simulink model "BMS_test"  (R2022b)
settings: Solver=FixedStepAuto  StartTime=0.0  StopTime=inf  FixedStep=0.005  RelTol=1e-3
undefined symbols (not defined in the file): canChannel
libraries: canlib x3, canmsglib x2, battery_monitor_lib x1
settings Model: Creator=LinF  LastModifiedBy=LinF

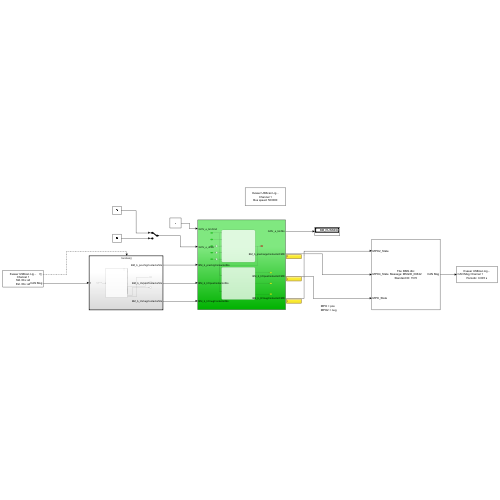
[thumbnail: Simulink's stored preview of the top-level diagram]
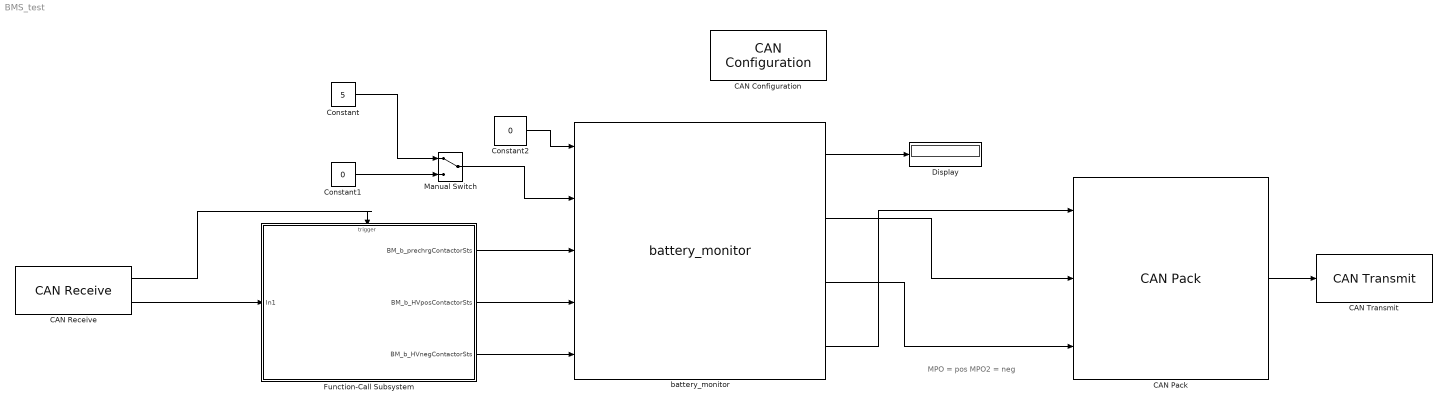
== system BMS_test ==
  note: MPO = pos
      | MPO2 = neg
  CAN Configuration : canlib/CAN Configuration  BlockHandle=2.0897  Device=Kvaser USBcan Light 1 (Channel 1)  DeviceMenu=Kvaser USBcan Light 1 (Channel 1)  ObjConstructor=canChannel('Kvaser', 'USBcan Light 1', 1)  BusSpeed=500000  EnableBitParameters=off  SJW=1  TSEG1=4  TSEG2=3  NSamples=1  AckMode=Normal
  CAN Pack : canmsglib/CAN Pack  CANdbFile=C:\Users\LinF\Documents\MACFE\Embedded\CAN_Databases\BMS.dbc  MsgList=MSGID_0X622  MsgName=MSGID_0X622  MsgIDType=Standard (11-bit identifier)  MsgIdentifier=1570  MsgLength=3  Remote=off  ApplyMinMax=off  BusOutput=off  SignalInfo={'MPO2_State','16','8','BE','unsigned','Standard','0','1','0','-Inf','Inf';'MPO4_State','8','8','BE','unsigned','Standard','0','1','0','-Inf','Inf';'MPO_State','0','8','BE','unsigned','Standard','0','1','0','-Inf','Inf'}
      settings: LibrarySourceBlock=embeddedtargetslib/Host Communication/CAN Pack  DataFormat=CANdb specified signals
  CAN Receive : canlib/CAN Receive  BlockHandle=8.0004  Device=Kvaser USBcan Light 1 (Channel 1)  DeviceMenu=Kvaser USBcan Light 1 (Channel 1)  ObjConstructor=canChannel('Kvaser', 'USBcan Light 1', 1)  EnableStandardIDsFilter=off  StdIDsCombo=Allow all  StandardIDs=0  EnableExtendedIDsFilter=off  ExtIDsCombo=Allow all  ExtendedIDs=0  SampleTime=0.005  MsgsPerTimestep=all  InternalFilterUpdateStatus=on  BusOutput=off
  CAN Transmit : canlib/CAN Transmit  BlockHandle=11.0004  Device=Kvaser USBcan Light 1 (Channel 1)  DeviceMenu=Kvaser USBcan Light 1 (Channel 1)  ObjConstructor=canChannel('Kvaser', 'USBcan Light 1', 1)  EnableEventTransmit=off  EnablePeriodicTransmit=on  MessagePeriod=0.005
  Constant : Constant  Value=5
  Constant1 : Constant  Value=0
  Constant2 : Constant  Value=0
  Display : Display
  Function-Call Subsystem : Subsystem  TreatAsAtomicUnit=on
  Manual Switch : ManualSwitch
  battery_monitor : battery_monitor_lib/battery_monitor  SystemSampleTime=-1  VariantActivationTime=update diagram  Latency=0  AutoFrameSizeCalculation=off
  wires:
  Manual Switch/1 -> battery_monitor/2
  Constant/1 -> Manual Switch/1
  Constant1/1 -> Manual Switch/2
  battery_monitor/1 -> Display/1
  Constant2/1 -> battery_monitor/1
  CAN Receive/2 -> Function-Call Subsystem/1(In1)
  CAN Receive/1 -> Function-Call Subsystem/Trigger
  battery_monitor/3 -> CAN Pack/3
  battery_monitor/4 -> CAN Pack/1
  battery_monitor/2 -> CAN Pack/2
  CAN Pack/1 -> CAN Transmit/1
  Function-Call Subsystem/1(BM_b_prechrgContactorSts) -> battery_monitor/3
  Function-Call Subsystem/2(BM_b_HVposContactorSts) -> battery_monitor/4
  Function-Call Subsystem/3(BM_b_HVnegContactorSts) -> battery_monitor/5

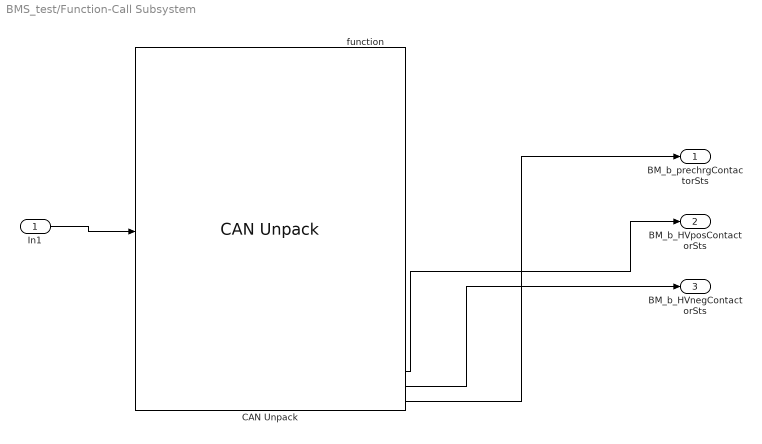
== system BMS_test/Function-Call Subsystem ==
  In1 : Inport
  function : TriggerPort  TriggerType=function-call  VariantControl=(inherit)
  CAN Unpack : canmsglib/CAN Unpack  CANdbFile=C:\Users\LinF\Documents\MACFE\Embedded\CAN_Databases\BMS.dbc  MsgList=MSGID_0X626  MsgName=MSGID_0X626  MsgIDType=Standard (11-bit identifier)  MsgIdentifier=1574  MsgLength=3  SignalInfo={'Blank','1','1','LE','unsigned','Standard','0','1','0','0','1';'Blank','2','1','LE','unsigned','Standard','0','1','0','0','1';'Blank','3','1','LE','unsigned','Standard','0','1','0','0','1';'Blank','4','1','LE','unsigned','Standard','0','1','0','0','1';'Blank','5','1','LE','unsigned','Standard','0','1','0','0','1';'Blank','6','1','LE','unsigned','Standard','0','1','0','0','1';'Blank','7','1','LE','unsigned','Standard','0','1','0','0','1';'Blank','9','1','LE','unsigned','Standard','0','1','0','0','1';'Blank','10','1','LE','unsigned','Standard','0','1','0','0','1';'Blank','11','1','LE','unsigned','Standard','0','1','0','0','1';'Blank','12','1','LE','unsigned','Standard','0','1','0','0','1';'Blank','13','1','LE','unsigned','Standard','0','1','0','0','1';'Blank','14','1','LE','unsigned','Standard','0','1','0','0','1';'Blank','15','1','LE','unsigned','Standard','0','1','0','0','1';'Blank','17','1','LE','unsigned','Standard','0','1','0','0','1';'Blank','18','1','LE','unsigned','Standard','0','1','0','0','1';'Blank','19','1','LE','unsigned','Standard','0','1','0','0','1';'Blank','20','1','LE','unsigned','Standard','0','1','0','0','1';'Blank','21','1','LE','unsigned','Standard','0','1','0','0','1';'Blank','22','1','LE','unsigned','Standard','0','1','0','0','1';'Blank','23','1','LE','unsigned','Standard','0','1','0','0','1';'MultiPurpose_Output','0','1','LE','unsigned','Standard','0','1','0','0','1';'MultiPurpose_Output_2','8','1','LE','unsigned','Standard','0','1','0','0','1';'MultiPurpose_Output_4','16','1','LE','unsigned','Standard','0','1','0','0','1'}  IDPort=off  TimestampPort=off  ErrorPort=off  RemotePort=off  LengthPort=off  StatusPort=off  ApplyMinMax=off
      settings: LibrarySourceBlock=canlib/CAN Unpack  DataFormat=CANdb specified signals
  BM_b_prechrgContactorSts : Outport
  BM_b_HVposContactorSts : Outport  Port=2
  BM_b_HVnegContactorSts : Outport  Port=3
  wires:
  In1/1 -> CAN Unpack/1
  CAN Unpack/24 -> BM_b_prechrgContactorSts/1
  CAN Unpack/22 -> BM_b_HVposContactorSts/1
  CAN Unpack/23 -> BM_b_HVnegContactorSts/1
